simulink model "Sobel_Edge_Detection_start"  (R2024a)
settings: Solver=VariableStepAuto  StartTime=0.0  StopTime=inf  RelTol=1e-3  EnableMultiTasking=on
libraries: hlsBasic x2, visionsinks x2, dspvision x1
settings Model: Creator=dvancamp  LastModifiedBy=robg
settings SolverCC: AlgebraicLoopSolver=TrustRegion
settings DataIOCC: LimitDataPoints=on  ReturnWorkspaceOutputs=off
settings OptimizationCC: LifeSpan=inf
settings DebuggingCC: InheritedTsInSrcMsg=none  UnconnectedInputMsg=warning  UnconnectedOutputMsg=warning  UnconnectedLineMsg=warning  AllowSymbolicDim=off  SFUnexpectedBacktrackingDiag=warning  SFNoUnconditionalDefaultTransitionDiag=warning  ArithmeticOperatorsInVariantConditions=warning
settings ModelReferenceCC: EnableRefExpFcnMdlSchedulingChecks=on  PropagateSignalLabelsOutOfModel=off
settings SFSimCC: SimUseLocalCustomCode=off  CustomCodeUndefinedFunction=UseInterfaceOnly
settings RTWCC: RTWUseLocalCustomCode=off  GPUComputeCapability=3.5
settings CodeAppCC: StateflowObjectComments=on
settings GRTTargetCC: TargetLangStandard=C89/C90 (ANSI)
settings ConfigComp: CovMetricSettings=dw  CovSaveCumulativeToWorkspaceVar=on  CovSaveSingleToWorkspaceVar=on  CovExternalEMLEnable=off  CovBoundaryAbsTol=1.0e-5

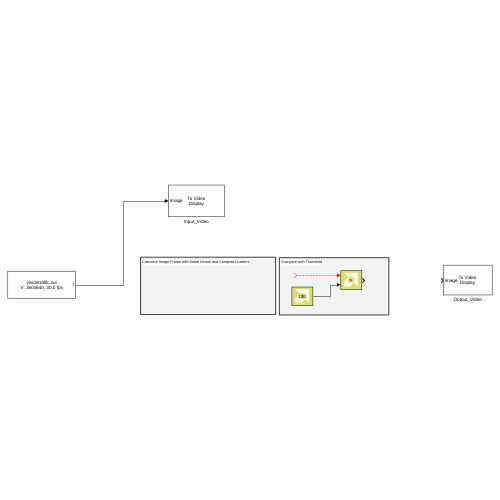
[thumbnail: Simulink's stored preview of the top-level diagram]
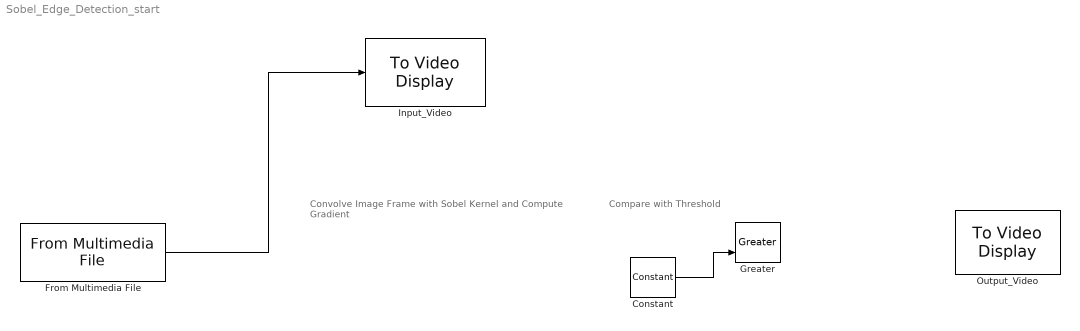
== system Sobel_Edge_Detection_start ==
  note: Compare with Threshold
  note: Convolve Image Frame with Sobel Kernel and Compute Gradient
  Constant : hlsBasic/Constant  Description=Performs multiplication  Value=130  VectorParams1D=off  SampleTime=-1  OutDataType=int16  TypeExp=''  Signedness=Signed  WordLength=16  FractionalLength=0  RoundingMode=Truncation to minus infinity  OverflowMode=Wrap around
  From Multimedia File : dspvision/From Multimedia File  inputFilename=visiontraffic.avi  readRange=[1 Inf]  loop=on  numPlays=inf  outputStreams=Video only  videoDataType=uint8  audioDataType=int16  inheritSampleTime=off  userDefinedSampleTime=1/30  noAudioOutput=off  isIntensityVideo=off  fourcc=Intensity  colorVideoFormat=One multidimensional signal  outputEOF=off  dataOrg=Column-major  audioFrameSize=1024  computeAudioFrameSize=off  outSamplingMode=Sample based
  Greater : hlsBasic/Greater  Description=Performs multiplication
  Input_Video : visionsinks/To Video Display  windowSizeMode=True size (1:1)  openAtMdlStart=on  fullScreen=off  videoWindowX=197  videoWindowY=628  saveWindowSize=off  videoWindowWidth=160  videoWindowHeight=120  inputColorFormat=RGB  inputType=Obsolete  imagePorts=One multidimensional signal  OutputDevice=On-screen video monitor  dataOrg=Column-major  isWindowOpen=off
  Output_Video : visionsinks/To Video Display  windowSizeMode=True size (1:1)  openAtMdlStart=on  fullScreen=off  videoWindowX=1115  videoWindowY=603  saveWindowSize=off  videoWindowWidth=640  videoWindowHeight=360  inputColorFormat=RGB  inputType=Obsolete  imagePorts=One multidimensional signal  OutputDevice=On-screen video monitor  dataOrg=Column-major  isWindowOpen=off
  wires:
  Constant/1 -> Greater/2
  ? -> Greater/1
  From Multimedia File/1 -> Input_Video/1
